simulink model "sim_rst"  (R2019b)
settings: Solver=VariableStepAuto  StartTime=0.0  StopTime=100  RelTol=1e-3
values from neighbouring files (symbols this model uses):
  a = [1 -1.0942 0.2800]    [calcul_rst.m]
  am = poly(am_root)    [calcul_rst.m]
  b = [0.0704]    [calcul_rst.m]
  bm = poly(bm_root)    [calcul_rst.m]
  r = [x(3:4)']    [calcul_rst.m]
  s = [1 x(2)]    [calcul_rst.m]
settings Model: Creator=ialex  LastModifiedBy=ialex

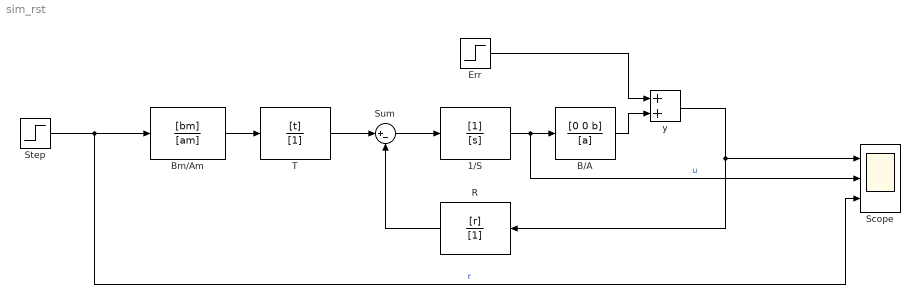
== system sim_rst ==
  1/S : DiscreteFilter  Denominator=[s]  FilterStructure=Direct form I
  B/A : DiscreteFilter  Numerator=[0 0 b]  Denominator=[a]  FilterStructure=Direct form I
  Bm/Am : DiscreteFilter  Numerator=[bm]  Denominator=[am]  FilterStructure=Direct form I
  Err : Step  Time=50  After=0.25  SampleTime=0
  R : DiscreteFilter  Numerator=[r]  Denominator=[1]  FilterStructure=Direct form I
  Scope : Scope  NumInputPorts=3
  Step : Step  SampleTime=0
  Sum : Sum  Inputs=|+-
  T : DiscreteFilter  Numerator=[t]  Denominator=[1]  FilterStructure=Direct form I
  y : Sum
  wires:
  Bm/Am/1 -> T/1
  T/1 -> Sum/1
  Sum/1 -> 1/S/1
  R/1 -> Sum/2
  B/A/1 -> y/2
  y/1 -> Scope/1, R/1
  Err/1 -> y/1
  1/S/1 -> Scope/2, B/A/1  "u"
  Step/1 -> Scope/3, Bm/Am/1  "r"
